simulink model "pomieszczenie"  (R2018b)
settings: Solver=ode45  StartTime=0.0  StopTime=10.0  MaxStep=maxstepsize  RelTol=1e-3
values from neighbouring files (symbols this model uses):
  cpw = 4175    [skrypt.m]
  Cv01 = cpw*row*Vv    (= 80160)    [skrypt.m]
  Cv02 = cpw*row*Vv    (= 80160)    [skrypt.m]
  Cvg1 = cpw*row*Vg1    (= 40080)    [skrypt.m]
  Cvg2 = cpw*row*Vg2    (= 40080)    [skrypt.m]
  Cvs1 = cps*ros*Vs1    (= 5665792)    [skrypt.m]
  Cvs2 = cps*ros*Vs2    (= 5665792)    [skrypt.m]
  Cvw1 = cpp*rop*Vw1    (= 48000)    [skrypt.m]
  Cvw2 = cpp*rop*Vw2    (= 48000)    [skrypt.m]
  dfmw = 0.2*fmw0    (= 0.00479041916168)    [skrypt.m]
  dTwew1_0 = 2    [identyfikacja transmitancji.m]    (also in skrypt.m = 0)
  dTwz = 0    [skrypt.m]
  dTzew = 0    [skrypt.m]
  fmg1_0 = fmg1_N    (= 0.0119760479042)    [skrypt.m]
  fmg2_0 = fmg2_N    (= 0.0119760479042)    [skrypt.m]
  fmw0 = fmwN    (= 0.0239520958084)    [skrypt.m]
  Kcg1 = qg1_N/(Tgp1_N-Twew1_N)    (= 20)    [skrypt.m]
  Kcg2 = qg2_N/(Tgp2_N-Twew2_N)    (= 19.2307692308)    [skrypt.m]
  Kco = qwN/(TwpN-TozN)    (= 100)    [skrypt.m]
  Kcs1 = qg1_N/(Ts1_N-TzewN)    (= 40)    [skrypt.m]
  Kcs2 = qg2_N/(Ts2_N-TzewN)    (= 41.6666666667)    [skrypt.m]
  Kcw1 = qg1_N/(Twew1_N-Ts1_N)    (= 66.6666666667)    [skrypt.m]
  Kcw2 = qg2_N/(Twew2_N-Ts2_N)    (= 71.4285714286)    [skrypt.m]
  ki = kp/Ti    (= 4.52196844658e-06)    [identyfikacja transmitancji.m]    (also in skrypt.m)
  kp = 0.9 * T3 /(k3*T30)    (= 0.173168781662)    [identyfikacja transmitancji.m]    (also in skrypt.m)
  L = [k3]    [identyfikacja transmitancji.m]
  M = [T3 ,1]    [identyfikacja transmitancji.m]
  steptime = czas*3*10^(-2)    (= 30000)    [skrypt.m]
  T30 = 11500    [identyfikacja transmitancji.m]    (also in skrypt.m)
  Tdelay1 = 3500    [skrypt.m]
  Tdelay2 = Tdelay1    (= 3500)    [skrypt.m]
  Tgp1_0 = (C_1*Tgz1_0+Kcg1*Twew1_0)/(Kcg1+C_1)    (= 70)    [skrypt.m]
  Tgp2_0 = (C_2*Tgz2_0+Kcg2*Twew2_0)/(Kcg2+C_2)    (= 70)    [skrypt.m]
  Toz0 = (Kco*C1*Twz0+C2*(C1+Kco)*Top0)/M_1    (= 90)    [skrypt.m]
  Ts1_0 = (Kcw1*Twew1_0+Kcs1*Tzew0)/(Kcw1+Kcs1)    (= 5)    [skrypt.m]
  Ts2_0 = (Kcw2*Twew2_0+Kcs2*Tzew0)/(Kcw2+Kcs2)    (= 4)    [skrypt.m]
  Twew1_0 = (Kcg1*C_1*(Kcw1+Kcs1)*Tgz1_0+Kcw1*Kcs1*(Kcg1+C_1)*Tzew0)/M_1    (= 20)    [skrypt.m]
  Twew2_0 = (Kcg2*C_2*(Kcw2+Kcs2)*Tgz2_0+Kcw2*Kcs2*(Kcg2+C_2)*Tzew0)/M_2    (= 18)    [skrypt.m]
  Twp0 = (C1*Twz0+Kco*Toz0)/(C1+Kco)    (= 110)    [skrypt.m]
  Twz0 = TwzN    (= 130)    [skrypt.m]
  Tzew0 = TzewN    (= -20)    [skrypt.m]
settings Model: Creator=LAB320-1552  LastModifiedBy=r3vus
settings DataIOCC: LimitDataPoints=on  SaveFormat=Array  SignalLoggingSaveFormat=ModelDataLogs
settings OptimizationCC: BlockReduction=off  BooleanDataType=off  LifeSpan=inf
settings DebuggingCC: SaveWithParameterizedLinksMsg=none  UnderspecifiedInitializationDetection=Classic  MergeDetectMultiDrivingBlocksExec=none  SignalResolutionControl=TryResolveAllWithWarning  MultiTaskDSMMsg=warning  MultiTaskCondExecSysMsg=none  StateNameClashWarn=warning  SFUnexpectedBacktrackingDiag=warning  SFNoUnconditionalDefaultTransitionDiag=warning  SFExecutionAtInitializationDiag=none
settings HardwareCC: ProdBitPerPointer=32  ProdBitPerSizeT=32  ProdBitPerPtrDiffT=32  ProdLargestAtomicFloat=None  ProdIntDivRoundTo=Undefined  ProdEndianess=Unspecified  ProdWordSize=32  ProdHWDeviceType=32-bit Generic  TargetUnknown=on
settings ModelReferenceCC: PropagateSignalLabelsOutOfModel=off
settings SFSimCC: SimUseLocalCustomCode=off
settings RTWCC: RTWUseLocalCustomCode=off
settings CodeAppCC: StateflowObjectComments=on
settings GRTTargetCC: TargetLangStandard=C89/C90 (ANSI)  GeneratePreprocessorConditionals=Disable all
settings ConfigComp: CovMetricSettings=dw  CovHtmlReporting=on  CovSaveCumulativeToWorkspaceVar=on  CovSaveSingleToWorkspaceVar=on  CovExternalEMLEnable=off

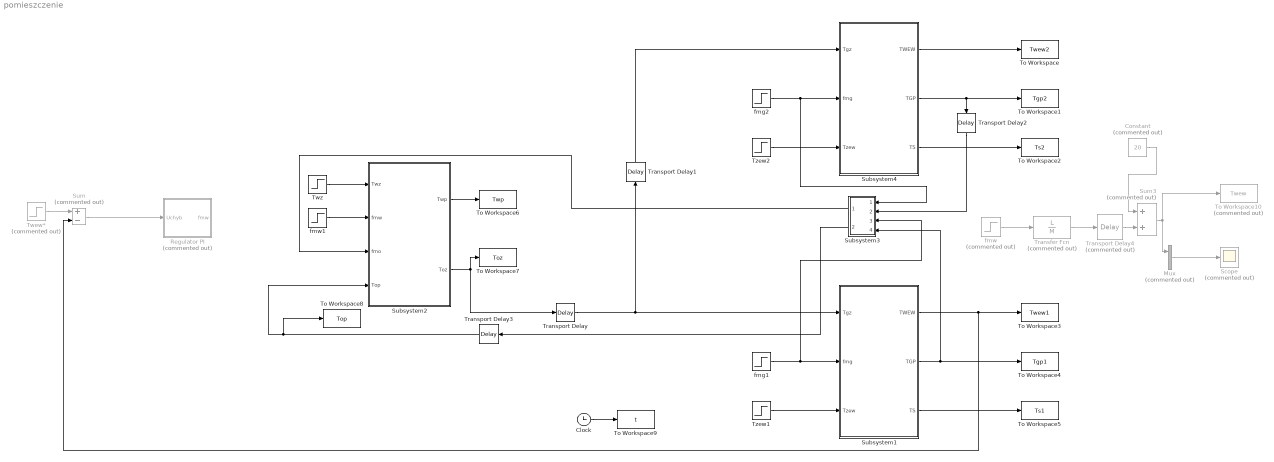
== system pomieszczenie ==
  Clock : Clock
  Constant : Constant  Commented=on  Value=20
  Mux : Mux  Commented=on  Inputs=2
  Regulator PI : Subsystem  Commented=on
  Scope : Scope  Commented=on
  Subsystem1 : Subsystem  mask{Kcg=Kcg1, Kcw=Kcw1, Cvw=Cvw1, Cvs=Cvs1, cpw=cpw, Kcs=Kcs1, Twew0=Twew1_0, Ts0=Ts1_0, Tgp0=Tgp1_0, Cvg=Cvg1}
  Subsystem2 : Subsystem  mask{cpw=cpw, Kco=Kco, Cv02=Cv02, Cv01=Cv01, Twp0=Twp0, Toz0=Toz0}
  Subsystem3 : Subsystem
  Subsystem4 : Subsystem  mask{Kcg=Kcg2, Kcw=Kcw2, Cvw=Cvw2, Cvs=Cvs2, cpw=cpw, Kcs=Kcs2, Twew0=Twew2_0, Ts0=Ts2_0, Tgp0=Tgp2_0, Cvg=Cvg2}
  Sum : Sum  Commented=on  Inputs=+-
  Sum3 : Sum  Commented=on
  To Workspace : ToWorkspace  VariableName=Twew2  SampleTime=-1
  To Workspace1 : ToWorkspace  VariableName=Tgp2  SampleTime=-1
  To Workspace10 : ToWorkspace  Commented=on  VariableName=Twew  SampleTime=-1
  To Workspace2 : ToWorkspace  VariableName=Ts2  SampleTime=-1
  To Workspace3 : ToWorkspace  VariableName=Twew1  SampleTime=-1
  To Workspace4 : ToWorkspace  VariableName=Tgp1  SampleTime=-1
  To Workspace5 : ToWorkspace  VariableName=Ts1  SampleTime=-1
  To Workspace6 : ToWorkspace  VariableName=Twp  SampleTime=-1
  To Workspace7 : ToWorkspace  VariableName=Toz  SampleTime=-1
  To Workspace8 : ToWorkspace  VariableName=Top  SampleTime=-1
  To Workspace9 : ToWorkspace  VariableName=t  SampleTime=-1
  Transfer Fcn : TransferFcn  Commented=on  Numerator=L  Denominator=M
  Transport Delay : TransportDelay  DelayTime=Tdelay1  InitialOutput=Toz0  BufferSize=10000
  Transport Delay1 : TransportDelay  DelayTime=Tdelay2  InitialOutput=Toz0  BufferSize=10000
  Transport Delay2 : TransportDelay  DelayTime=Tdelay2  InitialOutput=Tgp2_0  BufferSize=10000
  Transport Delay3 : TransportDelay  DelayTime=Tdelay1  InitialOutput=(Tgp1_0*fmg1_0+Tgp2_0*fmg2_0)/(fmg1_0+fmg2_0)  BufferSize=10000
  Transport Delay4 : TransportDelay  Commented=on  DelayTime=T30
  Twew* : Step  Commented=on  Time=steptime  Before=Twew1_0  After=Twew1_0+dTwew1_0  SampleTime=0
  Twz : Step  Time=steptime  Before=Twz0  After=Twz0+dTwz  SampleTime=0
  Tzew1 : Step  Time=steptime  Before=Tzew0  After=Tzew0+dTzew  SampleTime=0
  Tzew2 : Step  Time=steptime  Before=Tzew0  After=Tzew0+dTzew  SampleTime=0
  fmg1 : Step  Time=steptime  Before=fmg1_0  After=fmg1_0  SampleTime=0
  fmg2 : Step  Time=steptime  Before=fmg2_0  After=fmg2_0  SampleTime=0
  fmw : Step  Commented=on  Time=steptime  After=0+dfmw  SampleTime=0
  fmw1 : Step  Time=steptime  Before=fmw0  After=fmw0+dfmw  SampleTime=0
  wires:
  Subsystem2/2(Toz) -> Transport Delay/1, To Workspace7/1
  fmg2/1 -> Subsystem4/2(fmg), Subsystem3/1(fmg2)
  Tzew2/1 -> Subsystem4/3(Tzew)
  Subsystem4/1(TWEW) -> To Workspace/1
  Subsystem4/3(TS) -> To Workspace2/1
  Twz/1 -> Subsystem2/1(Twz)
  Subsystem2/1(Twp) -> To Workspace6/1
  fmg1/1 -> Subsystem1/2(fmg), Subsystem3/3(fmg1)
  Tzew1/1 -> Subsystem1/3(Tzew)
  Subsystem4/2(TGP) -> Transport Delay2/1, To Workspace1/1
  Subsystem1/3(TS) -> To Workspace5/1
  Subsystem1/2(TGP) -> Subsystem3/4(Tgp1), To Workspace4/1
  Transport Delay/1 -> Subsystem1/1(Tgz), Transport Delay1/1
  Transport Delay1/1 -> Subsystem4/1(Tgz)
  Transport Delay3/1 -> To Workspace8/1, Subsystem2/4(Top)
  Clock/1 -> To Workspace9/1
  Transport Delay2/1 -> Subsystem3/2(Tgp2)
  Subsystem3/1(fmo) -> Subsystem2/3(fmo)
  Subsystem3/2(top) -> Transport Delay3/1
  Twew*/1 -> Sum/1
  Sum/1 -> Regulator PI/1(Uchyb)
  Subsystem1/1(TWEW) -> Sum/2, To Workspace3/1
  Transfer Fcn/1 -> Transport Delay4/1
  fmw/1 -> Transfer Fcn/1
  Transport Delay4/1 -> Sum3/2
  Mux/1 -> Scope/1
  Constant/1 -> Sum3/1
  Sum3/1 -> Mux/1, To Workspace10/1
  fmw1/1 -> Subsystem2/2(fmw)

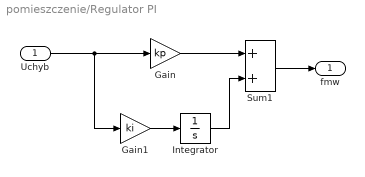
== system pomieszczenie/Regulator PI ==
  Uchyb : Inport
  Gain : Gain  Gain=kp
  Gain1 : Gain  Gain=ki
  Integrator : Integrator  InitialCondition=fmw0
  Sum1 : Sum
  fmw : Outport
  wires:
  Sum1/1 -> fmw/1
  Integrator/1 -> Sum1/2
  Gain1/1 -> Integrator/1
  Uchyb/1 -> Gain1/1, Gain/1
  Gain/1 -> Sum1/1

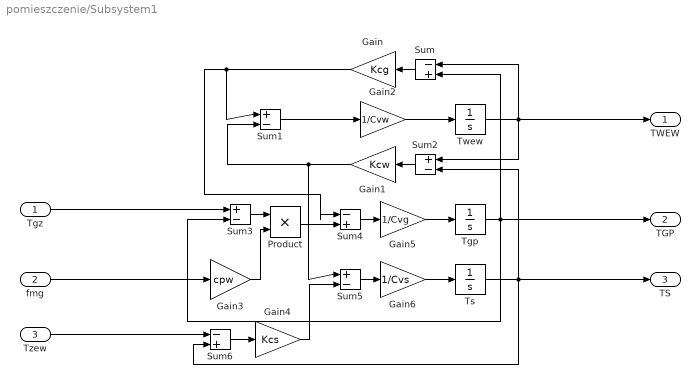
== system pomieszczenie/Subsystem1 ==
  Tgz : Inport
  fmg : Inport  Port=2
  Tzew : Inport  Port=3
  Gain : Gain  Gain=Kcg
  Gain1 : Gain  Gain=Kcw
  Gain2 : Gain  Gain=1/Cvw
  Gain3 : Gain  Gain=cpw
  Gain4 : Gain  Gain=Kcs
  Gain5 : Gain  Gain=1/Cvg
  Gain6 : Gain  Gain=1/Cvs
  Product : Product
  Sum : Sum  Inputs=-+
  Sum{1..3,5} (4 alike) : Sum  Inputs=+-
  Sum4 : Sum  Inputs=-+
  Sum6 : Sum  Inputs=-+
  Tgp : Integrator  InitialCondition=Tgp0
  Ts : Integrator  InitialCondition=Ts0
  Twew : Integrator  InitialCondition=Twew0
  TWEW : Outport
  TGP : Outport  Port=2
  TS : Outport  Port=3
  wires:
  Twew/1 -> TWEW/1, Sum2/1, Sum/1
  Tgp/1 -> TGP/1, Sum3/2, Sum/2
  Sum/1 -> Gain/1
  Ts/1 -> TS/1, Sum6/2, Sum2/2
  Sum2/1 -> Gain1/1
  Gain1/1 -> Sum5/1, Sum1/2
  Sum1/1 -> Gain2/1
  Tgz/1 -> Sum3/1
  fmg/1 -> Gain3/1
  Gain3/1 -> Product/2
  Sum3/1 -> Product/1
  Gain/1 -> Sum1/1, Sum4/1
  Product/1 -> Sum4/2
  Sum4/1 -> Gain5/1
  Tzew/1 -> Sum6/1
  Sum6/1 -> Gain4/1
  Gain4/1 -> Sum5/2
  Sum5/1 -> Gain6/1
  Gain2/1 -> Twew/1
  Gain5/1 -> Tgp/1
  Gain6/1 -> Ts/1

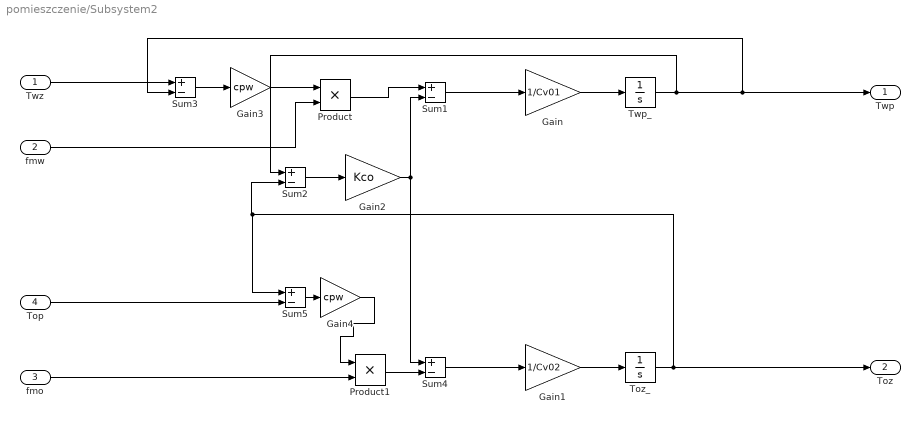
== system pomieszczenie/Subsystem2 ==
  Twz : Inport
  fmw : Inport  Port=2
  fmo : Inport  Port=3
  Top : Inport  Port=4
  Gain : Gain  Gain=1/Cv01
  Gain1 : Gain  Gain=1/Cv02
  Gain2 : Gain  Gain=Kco
  Gain3 : Gain  Gain=cpw
  Gain4 : Gain  Gain=cpw
  Product : Product
  Product1 : Product
  Sum{1..5} (5 alike) : Sum  Inputs=+-
  Toz_ : Integrator  InitialCondition=Toz0
  Twp_ : Integrator  InitialCondition=Twp0
  Twp : Outport
  Toz : Outport  Port=2
  wires:
  Toz_/1 -> Sum5/1, Sum2/2, Toz/1
  Twp_/1 -> Sum2/1, Sum3/2, Twp/1
  Gain/1 -> Twp_/1
  Gain1/1 -> Toz_/1
  Product/1 -> Sum1/1
  Sum1/1 -> Gain/1
  Sum2/1 -> Gain2/1
  Sum4/1 -> Gain1/1
  Gain2/1 -> Sum1/2, Sum4/1
  fmo/1 -> Product1/2
  Top/1 -> Sum5/2
  Product1/1 -> Sum4/2
  Twz/1 -> Sum3/1
  Sum3/1 -> Gain3/1
  Gain3/1 -> Product/1
  fmw/1 -> Product/2
  Sum5/1 -> Gain4/1
  Gain4/1 -> Product1/1

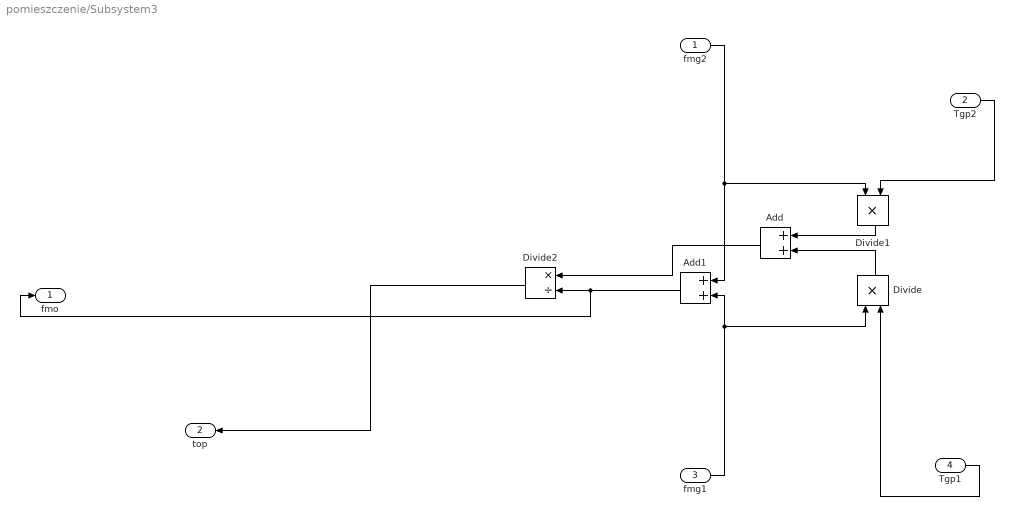
== system pomieszczenie/Subsystem3 ==
  fmg2 : Inport
  Tgp2 : Inport  Port=2
  fmg1 : Inport  Port=3
  Tgp1 : Inport  Port=4
  Add : Sum
  Add1 : Sum
  Divide : Product  Inputs=**
  Divide1 : Product  Inputs=**
  Divide2 : Product  Inputs=*/
  fmo : Outport
  top : Outport  Port=2
  wires:
  Divide1/1 -> Add/1
  Divide/1 -> Add/2
  fmg1/1 -> Add1/2, Divide/1
  Add1/1 -> fmo/1, Divide2/2
  fmg2/1 -> Add1/1, Divide1/1
  Add/1 -> Divide2/1
  Divide2/1 -> top/1
  Tgp1/1 -> Divide/2
  Tgp2/1 -> Divide1/2

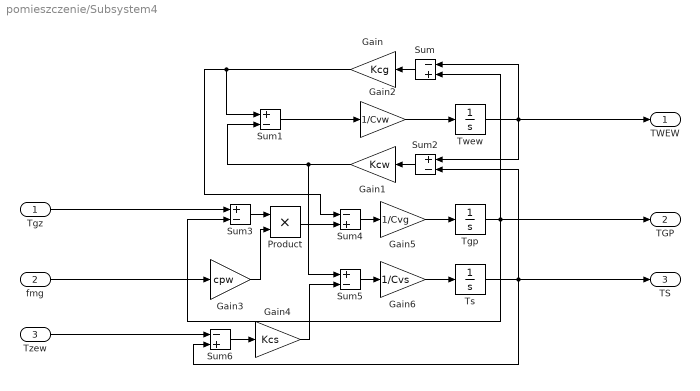
== system pomieszczenie/Subsystem4 ==
  Tgz : Inport
  fmg : Inport  Port=2
  Tzew : Inport  Port=3
  Gain : Gain  Gain=Kcg
  Gain1 : Gain  Gain=Kcw
  Gain2 : Gain  Gain=1/Cvw
  Gain3 : Gain  Gain=cpw
  Gain4 : Gain  Gain=Kcs
  Gain5 : Gain  Gain=1/Cvg
  Gain6 : Gain  Gain=1/Cvs
  Product : Product
  Sum : Sum  Inputs=-+
  Sum{1..3,5} (4 alike) : Sum  Inputs=+-
  Sum4 : Sum  Inputs=-+
  Sum6 : Sum  Inputs=-+
  Tgp : Integrator  InitialCondition=Tgp0
  Ts : Integrator  InitialCondition=Ts0
  Twew : Integrator  InitialCondition=Twew0
  TWEW : Outport
  TGP : Outport  Port=2
  TS : Outport  Port=3
  wires:
  Twew/1 -> TWEW/1, Sum2/1, Sum/1
  Tgp/1 -> TGP/1, Sum3/2, Sum/2
  Sum/1 -> Gain/1
  Ts/1 -> TS/1, Sum6/2, Sum2/2
  Sum2/1 -> Gain1/1
  Gain1/1 -> Sum5/1, Sum1/2
  Sum1/1 -> Gain2/1
  Tgz/1 -> Sum3/1
  fmg/1 -> Gain3/1
  Gain3/1 -> Product/2
  Sum3/1 -> Product/1
  Gain/1 -> Sum1/1, Sum4/1
  Product/1 -> Sum4/2
  Sum4/1 -> Gain5/1
  Tzew/1 -> Sum6/1
  Sum6/1 -> Gain4/1
  Gain4/1 -> Sum5/2
  Sum5/1 -> Gain6/1
  Gain2/1 -> Twew/1
  Gain5/1 -> Tgp/1
  Gain6/1 -> Ts/1
